simulink model "takeoff_real"  (R2024b)
settings: Solver=ode4  StartTime=0.0  StopTime=150  FixedStep=0.001  RelTol=1e-3
values from neighbouring files (symbols this model uses):
  a0 = 340.294    [basedata.m]    (also in basedata.mat; control_design.mat; landing_init.m; landing_plan.mat)
  b_ref = 2.0    (= 2)    [basedata.m]    (also in basedata.mat; control_design.mat; landing_init.m; landing_plan.mat)
  c_gear = [0.8e4, 1.4e4, 1.4e4]    [basedata.m]    (also in basedata.mat = [8000 14000 14000]; control_design.mat = [8000 14000 14000]; landing_init.m; landing_plan.mat = [8000 14000 14000])
  c_lat = [1.4e4, 2.2e4, 2.2e4]    [basedata.m]    (also in basedata.mat = [14000 22000 22000]; control_design.mat = [14000 22000 22000]; landing_init.m; landing_plan.mat = [14000 22000 22000])
  c_ref = 0.9    [basedata.m]    (also in basedata.mat; control_design.mat; landing_init.m; landing_plan.mat)
  c_roll = [0.020, 0.018, 0.018]    [basedata.m]    (also in basedata.mat = [0.02 0.018 0.018]; control_design.mat = [0.02 0.018 0.018]; landing_init.m; landing_plan.mat = [0.02 0.018 0.018])
  CD0 = 0.045    [basedata.m]    (also in basedata.mat; canshujisuan.m; control_design.mat; landing_init.m)
  CL0 = 0.083    [basedata.m]    (also in basedata.mat; control_design.mat; landing_init.m; landing_plan.mat)
  CLa = 3.80    (= 3.8)    [basedata.m]    (also in basedata.mat; canshujisuan.m = 2.5; control_design.mat; landing_init.m)
  Clb = -0.08    [basedata.m]    (also in basedata.mat; control_design.mat; landing_init.m; landing_plan.mat)
  Clda = -0.20    (= -0.2)    [basedata.m]    (also in basedata.mat; control_design.mat; landing_init.m; landing_plan.mat)
  CLde = 0.28    [basedata.m]    (also in basedata.mat; control_design.mat; landing_init.m; landing_plan.mat)
  Clp = -0.70    (= -0.7)    [basedata.m]    (also in basedata.mat; control_design.mat; landing_init.m; landing_plan.mat)
  CLq = 4.50    (= 4.5)    [basedata.m]    (also in basedata.mat; canshujisuan.m = 3; control_design.mat; landing_init.m)
  Clr = 0.08    [basedata.m]    (also in basedata.mat; control_design.mat; landing_init.m; landing_plan.mat)
  Cm0 = 0.060    (= 0.06)    [basedata.m]    (also in basedata.mat; control_design.mat; landing_init.m; landing_plan.mat)
  Cma = -0.80    (= -0.8)    [basedata.m]    (also in basedata.mat; control_design.mat; landing_init.m; landing_plan.mat)
  Cmde = -0.90    (= -0.9)    [basedata.m]    (also in basedata.mat; control_design.mat; landing_init.m; landing_plan.mat)
  Cmq = -18.0    (= -18)    [basedata.m]    (also in basedata.mat; control_design.mat; landing_init.m; landing_plan.mat)
  Cnb = 0.25    [basedata.m]    (also in basedata.mat; control_design.mat; landing_init.m; landing_plan.mat)
  Cndr = -0.15    [basedata.m]    (also in basedata.mat; control_design.mat; landing_init.m; landing_plan.mat)
  Cnp = -0.04    [basedata.m]    (also in basedata.mat; control_design.mat; landing_init.m; landing_plan.mat)
  Cnr = -0.45    [basedata.m]    (also in basedata.mat; control_design.mat; landing_init.m; landing_plan.mat)
  CSb = -0.70    (= -0.7)    [basedata.m]    (also in basedata.mat; control_design.mat; landing_init.m; landing_plan.mat)
  CSdr = 0.18    [basedata.m]    (also in basedata.mat; control_design.mat; landing_init.m; landing_plan.mat)
  CSr = 0.12    [basedata.m]    (also in basedata.mat; control_design.mat; landing_init.m; landing_plan.mat)
  D = 0.5 * rho0 * V^2 * S_ref * CD_current    [canshujisuan.m]
  D0 = 1400    [basedata.m]    (also in basedata.mat; control_design.mat = 800; landing.m; landing_init.m)
  da_max = 25    [basedata.m]    (also in basedata.mat; control_design.mat; landing_init.m; landing_plan.mat)
  da_min = -da_max    (= -25)    [basedata.m]    (also in basedata.mat; control_design.mat; landing_init.m; landing_plan.mat)
  de_max = 25    [basedata.m]    (also in basedata.mat; control_design.mat; landing_init.m; landing_plan.mat)
  de_min = -de_max    (= -25)    [basedata.m]    (also in basedata.mat; control_design.mat; landing_init.m; landing_plan.mat)
  DH = pi / 180    (= 0.0174532925199)    [basedata.m]    (also in basedata.mat; control_design.mat; landing_init.m; landing_plan.mat)
  dr_max = 25    [basedata.m]    (also in basedata.mat; control_design.mat; landing_init.m; landing_plan.mat)
  dr_min = -dr_max    (= -25)    [basedata.m]    (also in basedata.mat; control_design.mat; landing_init.m; landing_plan.mat)
  g = 9.80665    [basedata.m]    (also in basedata.mat; canshujisuan.m; control_design.mat; landing_init.m)
  gamma1 = -0.125844364415    [basedata.mat]    (also in landing_trajectory.m = asin(max(min(gamma1_arg, 1), -1)); landingplan.mat)
  gamma2 = -0.0261780104712    [basedata.mat]    (also in landing_trajectory.m = -0.0261799387799; landingplan.mat = 0.0261780104712)
  ground_z = 0.0    (= 0)    [basedata.m]    (also in basedata.mat; control_design.mat; landing_init.m; landing_plan.mat)
  HD = 180 / pi    (= 57.2957795131)    [basedata.m]    (also in basedata.mat; control_design.mat; landing_init.m; landing_plan.mat)
  I = [ Ixx, -Ixy, -Ixz ... (first row only)    [basedata.m]    (also in basedata.mat = [120  0  0; 0  480  0; 0  0  520]; control_design.mat = [120  0  0; 0  480  0; 0  0  520]; landing_init.m; landing_plan.mat = [120  0  0; 0  480  0; 0  0  520])
  K = 0.12    [basedata.m]    (also in basedata.mat; canshujisuan.m = 0.08; control_design.mat; landing_init.m)
  K_alpha = 7.5375    [basedata.mat]    (also in control_design.m = (((wd_pitch^2)-a24))/(2*kesi_pitch*wd_pitch); control_design.mat; controller.m = 5; landingplan.mat)
  k_gear = [1.0e5, 3.0e5, 3.0e5]    [basedata.m]    (also in basedata.mat = [100000 300000 300000]; control_design.mat = [100000 300000 300000]; landing_init.m; landing_plan.mat = [100000 300000 300000])
  Kn_pitch = -0.120095403309    [basedata.mat]    (also in control_design.m = -(2.2*g*(wd_pitch)^2)/(Tr*(((wd_pitch)^2)-a24)*V_control*a34; control_design.mat; controller.m = (2.2*wd^2*g)/(Tr*(wd^2-a24)*V_test*a34); landingplan.mat)
  Kw_pitch = -0.483749055178    [basedata.mat]    (also in control_design.m = -2*kesi_pitch*wd_pitch/a25; control_design.mat; controller.m = -(2*zeta*wd) / a25; landingplan.mat)
  m = 600.0    (= 600)    [basedata.m]    (also in basedata.mat; canshujisuan.m; control_design.mat; landing_init.m)
  mu_brake = [0.0, 0.55, 0.55]    [basedata.m]    (also in basedata.mat = [0 0.55 0.55]; control_design.mat = [0 0.55 0.55]; landing_init.m; landing_plan.mat = [0 0.55 0.55])
  phi0 = 0    [control_design.mat]    (also in landing.m; landing_init.m; landing_init.mat; landing_plan.mat)
  psi0 = 0    [control_design.mat]    (also in landing.m; landing_init.m; landing_init.mat; landing_plan.mat)
  r_left_b = r_gear_b(:,2)    [basedata.m]    (also in basedata.mat = [-0.333333333333 -0.8 0.65]; control_design.mat = [-0.333333333333 -0.8 0.65]; landing_init.m; landing_plan.mat = [-0.333333333333 -0.8 0.65])
  r_nose_b = r_gear_b(:,1)    [basedata.m]    (also in basedata.mat = [2 0 0.65]; control_design.mat = [2 0 0.65]; landing_init.m; landing_plan.mat = [2 0 0.65])
  r_right_b = r_gear_b(:,3)    [basedata.m]    (also in basedata.mat = [-0.333333333333 0.8 0.65]; control_design.mat = [-0.333333333333 0.8 0.65]; landing_init.m; landing_plan.mat = [-0.333333333333 0.8 0.65])
  rho0 = 1.225    [basedata.m]    (also in basedata.mat; canshujisuan.m; control_design.mat; landing_init.m)
  S_ref = 1.2    [basedata.m]    (also in basedata.mat; canshujisuan.m; control_design.mat; landing_init.m)
  theta0 = 0    [control_design.mat]    (also in landing.m; landing_init.m; landing_init.mat = 0.0523598775598; landing_plan.mat = 0.0523560209424)
  u0_b = 0    [control_design.mat]    (also in landing.m = 128; landing_init.m = 128; landing_init.mat = 100; landing_plan.mat = 128)
  v0_b = 0    [control_design.mat]    (also in landing.m; landing_init.m; landing_init.mat; landing_plan.mat)
  V_app = 128.516392565    [basedata.mat]    (also in landing_trajectory.m = 1.4 * Vs; landingplan.mat)
  v_eps = 0.20    (= 0.2)    [basedata.m]    (also in basedata.mat; control_design.mat; landing_init.m; landing_plan.mat)
  V_flare = V_shallow    [landing_trajectory.m]
  V_min = 3    [control_design.mat]    (also in landing.m; landing_init.m; landing_plan.mat; landingplan.mat)
  V_shallow = 110.156907913    [basedata.mat]    (also in landing_trajectory.m = 1.2 * Vs; landingplan.mat)
  w0_b = 0    [control_design.mat]    (also in landing.m; landing_init.m; landing_init.mat; landing_plan.mat)
  wheel_radius = 0.18    [basedata.m]    (also in basedata.mat; control_design.mat; landing_init.m; landing_plan.mat)
  WOW_on = 0.000    (= 0)    [basedata.m]    (also in basedata.mat; control_design.mat; landing_init.m; landing_plan.mat)
  X_B = -4048.29417932    [basedata.mat]    (also in landing_trajectory.m = X_R - R * sin(a1); landingplan.mat)
  X_C = -3253.59462264    [basedata.mat]    (also in landing_trajectory.m = X_R - R * sin(a2); landingplan.mat)
  X_D = -1263.82547196    [basedata.mat]    (also in landing_trajectory.m = X_aim - H_exp / tan(a2); landingplan.mat)
  X_entry = -10904.3307826    [basedata.mat]    (also in landing_trajectory.m = X_zero - H_entry / tan(a1); landingplan.mat)
  Xg0 = 0    [control_design.mat]    (also in landing.m = -12000; landing_init.m = -12000; landing_init.mat = -8000; landing_plan.mat = -12000)
  Yg0 = 3    [control_design.mat]    (also in landing.m = 0; landing_init.m = 0; landing_init.mat = 0; landing_plan.mat = 0)
  Zg0 = ground_z - wheel_radius - r_gear_b(3,1) + static_deflection    [basedata.m]    (also in basedata.mat = -0.8215943; control_design.mat = -0.8215943; landing.m = -1000; landing_init.m = -1000)
undefined symbols (not defined in the file or in its folder): I_xz, I_yz, Ix_Iy, Iy_Iz, Iz_Ix
libraries: simulink x66, matrix_library x19
(part 4 of 4)

== matlab function takeoff_real/6DOF-MODEL/动力学/height/MATLAB Function1 ==
  data: phi input; R_bg output; theta input; psi input
function R_bg = ground2body(phi, theta, psi)
T1 = [cos(psi), sin(psi), 0;
     -sin(psi), cos(psi), 0;
      0, 0, 1];
T2 = [cos(theta), 0, -sin(theta);
       0, 1, 0;
      sin(theta), 0, cos(theta)];
T3 = [1, 0, 0;
      0, cos(phi), sin(phi);
      0, -sin(phi), cos(phi)];
R_bg = T3 * T2 * T1;

== matlab function takeoff_real/Guidance/4_拉平制导/MATLAB Function1 ==
  data: Flight_Phase input; Vxg input; gamma_cmd output; X_pos input
function gamma_cmd = flare_gamma_cmd(Flight_Phase, Vxg, X_pos)
%#codegen
% phase11 只做拉平段航迹角指令
% gamma_cmd: rad，下降为负
% 不包含接地段，不指令高度到 0

FLARE_PHASE = uint8(11);

X_D = -1601.388;     % 拉平开始位置, m
H0 = 20.0;           % 拉平开始高度, m
H_flare_end = 3.0;   % 拉平结束高度, m，接地段从这里以后接管
sigma = 8.5;         % 拉平时间常数, s

if Flight_Phase == FLARE_PHASE

    % 用位置计算进入拉平后的等效时间，避免 persistent 报连续采样时间错误
    V_use = max(abs(Vxg), 1.0);
    tau = max((X_pos - X_D) / V_use, 0.0);

    % 只拉平到 H_flare_end，不算到地面
    Hdot_cmd = -((H0 - H_flare_end) / sigma) * exp(-tau / sigma);

    % 高度变化率转航迹角
    s = Hdot_cmd / V_use;

    % 拉平段下滑角限制：只允许负值，且不要太陡
    s = min(max(s, -0.08), 0.0);

    gamma_cmd = asin(s);

else
    gamma_cmd = 0.0;
end

== stateflow chart takeoff_real/Flight Phase Manager/Phase Logic ==
  state Takeoff_Mode
    state Ground_Roll
      en: Flight_Phase = 1;
    state Rotation
      en: Flight_Phase = 2;
    state Liftoff
      en: Flight_Phase = 3;
    state Initial_Climb
      en: Flight_Phase = 4;
    state Climb_Complete
      en: Flight_Phase = 5;
    (default) -> Ground_Roll
    Rotation -> Liftoff : [airborne == true]
    Ground_Roll -> Rotation : [reach_VR==true]
    Liftoff -> Initial_Climb : [safe_climb == true]
    Initial_Climb -> Climb_Complete : [h_AGL  >= 800.0]
  state Landing_Mode
    state Glideslope_Capture
      en: Flight_Phase = 7;
    state Glideslope_Track
      en: Flight_Phase = 8;
    state Round_Flare
      en: Flight_Phase = 9;
    state Approach_Turn
      en: Flight_Phase = 6;
    state Roll_out
      en: Flight_Phase = 13;
    state Touchdown
      en: Flight_Phase = 12;
    state Flare
      en: Flight_Phase = 11;
    state Shallow_Glide
      en: Flight_Phase = 10;
    (default) -> Approach_Turn
    Approach_Turn -> Glideslope_Capture : [localizer_captured == true]
    Glideslope_Track -> Round_Flare : [in_round==true]
    Glideslope_Capture -> Glideslope_Track : [glideslope_captured == true]
    Round_Flare -> Shallow_Glide : [Slight_decline==true]
    Touchdown -> Roll_out : [nose_on_ground == true && V_runway < 35.0]
    Flare -> Touchdown : [main_on_ground == true]
    Shallow_Glide -> Flare : [in_Flare==true]
  (junction 38) -> Takeoff_Mode [order 1] : [Task_Mode == 1]{Flight_Phase = 0;}
  (default) -> (junction 38)
  (junction 38) -> Landing_Mode [order 2] : {Flight_Phase = 0;}
  data: h_AGL input size=1; V_runway input size=1; h_dot input; nose_on_ground input size=1; main_on_ground input size=1; airborne input size=1; reach_VR input size=1; safe_climb input size=1; localizer_captured input size=1; glideslope_captured input size=1; flare_entry input size=1; stop_condition input size=1; Task_Mode input size=1; Flight_Phase output uint8 size=1 =0; in_round input; in_Flare input; Slight_decline input

== matlab function takeoff_real/Guidance/1_地面制导/MATLAB Function ==
  data: Flight_Phase input; gamma_cmd output; Vxg input; h_AGL input
function gamma_cmd = touchdown_gamma_cmd(Flight_Phase, Vxg, h_AGL)
%#codegen
% phase12 接地段航迹角指令
% gamma_cmd: rad，下降为负
% 拉平段结束后由该函数接管

TOUCH_PHASE = uint8(12);

H_touch = 0.15;       % 判定接地附近高度, m
V_sink_td = 0.30;     % 接地段期望下沉率, m/s
V_sink_max = 0.45;    % 最大允许下沉率, m/s

if Flight_Phase == TOUCH_PHASE

    h = max(h_AGL, 0.0);
    V_use = max(abs(Vxg), 1.0);

    if h <= H_touch
        % 已到接地附近，航迹角指令归零，后面交给地面滑跑/接地控制
        Hdot_cmd = 0.0;
    else
        % 接地段：保持小下沉率，不再继续拉平
        Hdot_cmd = -V_sink_td;

        % 限制最大下沉率
        if Hdot_cmd < -V_sink_max
            Hdot_cmd = -V_sink_max;
        end
    end

    s = Hdot_cmd / V_use;

    % 接地段航迹角很小，避免给过大低头指令
    s = min(max(s, -0.02), 0.0);

    gamma_cmd = asin(s);

else
    gamma_cmd = 0.0;
end

== matlab function takeoff_real/6DOF-MODEL/动力学/起落架模型/纵向力/Subsystem/MATLAB Function ==
  data: phi input; R_bg output; theta input; psi input
function R_bg = ground2body(phi, theta, psi)
T1 = [cos(psi), sin(psi), 0;
     -sin(psi), cos(psi), 0;
      0, 0, 1];
T2 = [cos(theta), 0, -sin(theta);
       0, 1, 0;
      sin(theta), 0, cos(theta)];
T3 = [1, 0, 0;
      0, cos(phi), sin(phi);
      0, -sin(phi), cos(phi)];
R_bg = T3 * T2 * T1;

== matlab function takeoff_real/6DOF-MODEL/动力学/起落架模型/纵向力/Subsystem/主轮滚动方向向量 ==
  data: Cbg input; eg_long output; eb_long input
function eg_long = project_long(Cbg, eb_long)

e_z = [0; 0; 1];              % 前-右-下坐标系：Z 轴向下
P_g = eye(3) - e_z*e_z.';     % 投影到地面水平面

eg_long = P_g * Cbg * eb_long;

n = norm(eg_long);
if n > 1e-8
    eg_long = eg_long / n;
else
    eg_long = [1; 0; 0];
end

== matlab function takeoff_real/6DOF-MODEL/动力学/起落架模型/纵向力/Subsystem/前轮滚动方向向量 ==
  data: Cbg input; eg_long output; eb_long input
function eg_long = project_long(Cbg, eb_long)

e_z = [0; 0; 1];              % 前-右-下坐标系中，Z 轴为下
P_g = eye(3) - e_z*e_z.';     % 投影到地面水平面

eg_long = P_g * Cbg * eb_long;

n = norm(eg_long);
if n > 1e-8
    eg_long = eg_long / n;
else
    eg_long = [1; 0; 0];
end

== matlab function takeoff_real/6DOF-MODEL/动力学/起落架模型/起落架三轮质心在地系下位置/MATLAB Function ==
  data: phi input; R_bg output; theta input; psi input
function R_bg = ground2body(phi, theta, psi)
T1 = [cos(psi), sin(psi), 0;
     -sin(psi), cos(psi), 0;
      0, 0, 1];
T2 = [cos(theta), 0, -sin(theta);
       0, 1, 0;
      sin(theta), 0, cos(theta)];
T3 = [1, 0, 0;
      0, cos(phi), sin(phi);
      0, -sin(phi), cos(phi)];
R_bg = T3 * T2 * T1;
